simulink library "Power_Electric3Motor"  (R2018b)
settings: Solver=VariableStepAuto  StartTime=0.0  StopTime=10.0  RelTol=1e-3
undefined symbols (not defined in the file): ShaftF, ShaftRL, ShaftRR, VDatabase
libraries: fl_lib x4, Power_Components x3, elec_lib x2, nesl_utility x1, sm_lib x1, Cooling_3_Motor x1
Description:
  | Component of Simscape Vehicle Templates Library
  | 
  | Copyright 2018-2020 The MathWorks, Inc.
settings Model: Creator=smiller  LastModifiedBy=smiller

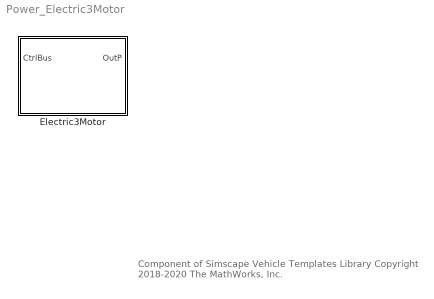
== system Power_Electric3Motor ==
  note: Component of Simscape Vehicle Templates Library
      | Copyright 2018-2020 The MathWorks, Inc.
  Electric3Motor : Subsystem  mask(Electric Propulsion with Three Motors){Power=VDatabase.Power.Electric3Motor_default, InitTriggerDropdown=0}
      mask prompts: Power "Power 3 Motor (structure)"; InitTriggerDropdown "Initialization Trigger Dropdown"
      mask help: Three electric motors with optional cooling system. Physical connections for the three motor shafts are in bus Shafts.
      mask init:
      | curblk = gcb;
      | 
      | % Trigger Mask Initialization for 
      | % variant subsystems below this level
      | sm_car_lib_maskInitTrigger(curblk)
      mask TypeOptions InitTriggerDropdown: 0 | 1
      mask Display: image('sm_car_vehicle_power_e3motor_IMAGE.png');

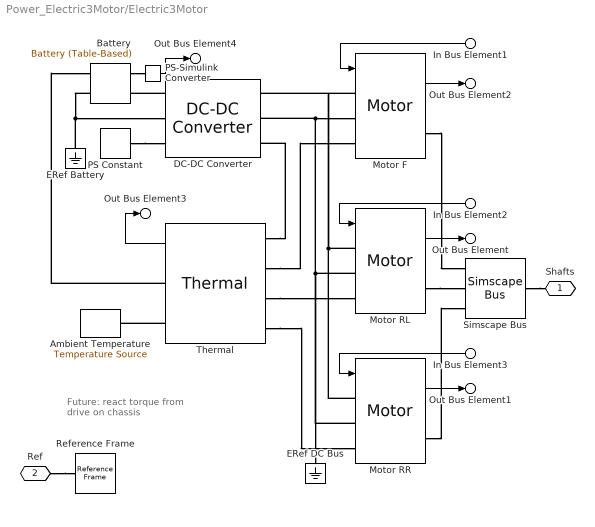
== system Power_Electric3Motor/Electric3Motor ==
  note: Future:
      | react torque
      | from drive
      | on chassis
  In Bus Element1 : Inport  PortName=CtrlBus  Element=MMotorFDemand
  In Bus Element2 : Inport  PortName=CtrlBus  Element=MMotorRLDemand
  In Bus Element3 : Inport  PortName=CtrlBus  Element=MMotorRRDemand
  Ambient Temperature : fl_lib/Thermal/Thermal Sources/Temperature Source  temperature=Power.TAmbient.Value K
      settings: SourceProductName=Simscape
  Battery : elec_lib/Sources/Battery (Table-Based)  SOC_vec=Power.Battery.vNoLoad.SOC.Value  T_vec=Power.Battery.vNoLoad.T.Value K  V0_mat=Power.Battery.vNoLoad.V0.Value V  R0_mat=Power.Battery.rTerminal.R0.Value Ohm  AH_vec=Power.Battery.AhTable.Ah.Value hr*A  prm_leak=1  Rleak_vec=[8000, 7000, 6000] Ohm  prm_dyn=1  R1_mat=[.089, .076, .01; .042, .022, .099; .019, .007, .002; .051, .043, .029] Ohm  tau1_mat=[44, 148, 235; 93, 110, 1000; 19, 27, 133; .5, 22, 3] s  R2_mat=[.014, .382, .407; .028, .006, .007; .014, .007, .006; .333, .956, .912] Ohm  tau2_mat=[1, 44, 5644; 11, 24, 506; 2, 14, 330; 3310, 13419, 30216] s  R3_mat=[.014, .382, .407; .028, .006, .007; .014, .007, .006; .333, .956, .912] Ohm  tau3_mat=[1, 44, 5644; 11, 24, 506; 2, 14, 330; 3310, 13419, 30216] s  R4_mat=[.014, .382, .407; .028, .006, .007; .014, .007, .006; .333, .956, .912] Ohm  tau4_mat=[1, 44, 5644; 11, 24, 506; 2, 14, 330; 3310, 13419, 30216] s  R5_mat=[.014, .382, .407; .028, .006, .007; .014, .007, .006; .333, .956, .912] Ohm  tau5_mat=[1, 44, 5644; 11, 24, 506; 2, 14, 330; 3310, 13419, 30216] s  N0=100  dV0=0  dR0=0  dAH=0  dRleak=0  dR1=0  dR2=0  dR3=0  dR4=0  dR5=0  temperature=300 K  i_specify=off  i_priority=None  i=0 A  i_nominal_specify=off  i_nominal_unit=A  i_nominal_value=1  v_specify=off  v_priority=None  v=0 V  v_nominal_specify=off  v_nominal_unit=V  v_nominal_value=1  stateOfCharge_specify=on  stateOfCharge_priority=High  stateOfCharge=Power.Battery.SOCInit.Value  stateOfCharge_nominal_specify=off  stateOfCharge_nominal_unit=1  stateOfCharge_nominal_value=1  num_cycles_specify=off  num_cycles_priority=High  num_cycles=0  num_cycles_nominal_specify=off  num_cycles_nominal_unit=1  num_cycles_nominal_value=1  thermal_mass=30000 J/K  temperature_specify=on  temperature_priority=High  temperature_nominal_specify=off  temperature_nominal_unit=K  temperature_nominal_value=1
      settings: SourceProductName=Simscape Electronics  SourceProductBaseCode=SN
  DC-DC Converter : elec_lib/Sources/DC-DC Converter  v_ref=Power.Converter.vRef.Value V  P_rated=Power.Converter.Power.Value W  droop_param=1  droop=0.001*0 V/A  droop_percent=2  reversible=1  efficiency=Power.Converter.efficiency.Value  P_fixed=1 W  model_dynamics=1  tau=Power.Converter.fConverter.Value s  v_ini=Power.Converter.vRef.Value V  G_diode=1e-8 1/Ohm  i1_max=Power.Converter.iMaxSupply.Value A  fault_condition=1  fault_threshold=0.5  thermal_mass=500 J/K  initial_temperature=25 degC
      settings: SourceProductName=Simscape Electronics  SourceProductBaseCode=SN
  ERef Battery : fl_lib/Electrical/Electrical Elements/Electrical Reference
  ERef DC Bus : fl_lib/Electrical/Electrical Elements/Electrical Reference
  Motor F : Power_Components/Motor  Motor=Power.MotorRR
  Motor RL : Power_Components/Motor  Motor=Power.MotorRL
  Motor RR : Power_Components/Motor  Motor=Power.MotorRR
  PS Constant : fl_lib/Physical Signals/Sources/PS Constant  constant=0
  PS-Simulink Converter : nesl_utility/PS-Simulink Converter  PhysicalDomain=network_engine_domain  SubClassName=ps_output  LeftPortType=input  RightPortType=output  PseudoPeriodic=off  Frequencies=[]  Unit=1  AffineConversion=off
  Reference Frame : sm_lib/Frames and Transforms/Reference Frame
  Simscape Bus : SimscapeBus  HierarchyStrings=ShaftF;ShaftRL;ShaftRR
  Thermal : Cooling_3_Motor/Thermal  VariantControl=Variant1  LabelModeActiveChoice=None  VariantLabel=Power.Cooling.class.Value  InitTriggerDropdown=0
      settings: AttributesFormatString=%<ActiveVariant>
  Shafts : PMIOPort  Side=Left
  Ref : PMIOPort  Port=2  Side=Right
  Out Bus Element : Outport  PortName=OutP  Element=MotorRL
  Out Bus Element1 : Outport  PortName=OutP  Element=MotorRR
  Out Bus Element2 : Outport  PortName=OutP  Element=MotorF
  Out Bus Element3 : Outport  PortName=OutP  Element=Thermal
  Out Bus Element4 : Outport  PortName=OutP  Element=BatterySOC
  wires:
  In Bus Element2/1 -> Motor RL/1
  In Bus Element1/1 -> Motor F/1
  Motor RL/1 -> Out Bus Element/1
  Motor RR/1 -> Out Bus Element1/1
  Motor F/1 -> Out Bus Element2/1
  In Bus Element3/1 -> Motor RR/1
  Thermal/1 -> Out Bus Element3/1
  PS-Simulink Converter/1 -> Out Bus Element4/1
  connections:
  Battery/LConn2 -- PS-Simulink Converter/LConn1
  PS Constant/RConn1 -- DC-DC Converter/LConn3
  DC-DC Converter/LConn1 -- Battery/LConn1
  Motor RR/RConn1 -- Simscape Bus/LConn3
  ERef Battery/LConn1 -- Battery/RConn1 -- DC-DC Converter/LConn2
  Motor RL/LConn2 -- Motor RR/LConn2 -- ERef DC Bus/LConn1 -- Motor F/LConn2 -- DC-DC Converter/RConn2
  Motor RL/LConn1 -- Motor RR/LConn1 -- Motor F/LConn1 -- DC-DC Converter/RConn1
  Motor F/RConn1 -- Simscape Bus/LConn1
  Motor RL/RConn1 -- Simscape Bus/LConn2
  Simscape Bus/RConn1 -- Shafts/RConn1
  Ref/RConn1 -- Reference Frame/RConn1
  Thermal/LConn1 -- DC-DC Converter/RConn3
  Thermal/LConn2 -- Motor F/LConn3
  Thermal/LConn3 -- Motor RL/LConn3
  Thermal/LConn4 -- Motor RR/LConn3
  Thermal/RConn1 -- Battery/RConn2
  Thermal/RConn2 -- Ambient Temperature/LConn1
